simulink model "Vnernst"  (R2023a)
settings: Solver=VariableStepAuto  StartTime=0.0  StopTime=10.0  RelTol=1e-3
undefined symbols (not defined in the file): F, K, Kr, R, Uopt
settings Model: Creator=meghn  LastModifiedBy=meghn

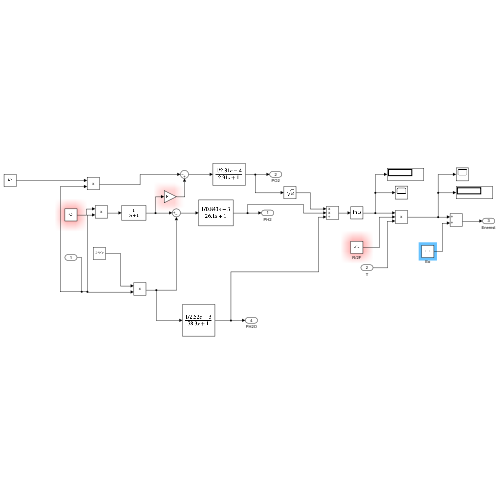
[thumbnail: Simulink's stored preview of the top-level diagram]
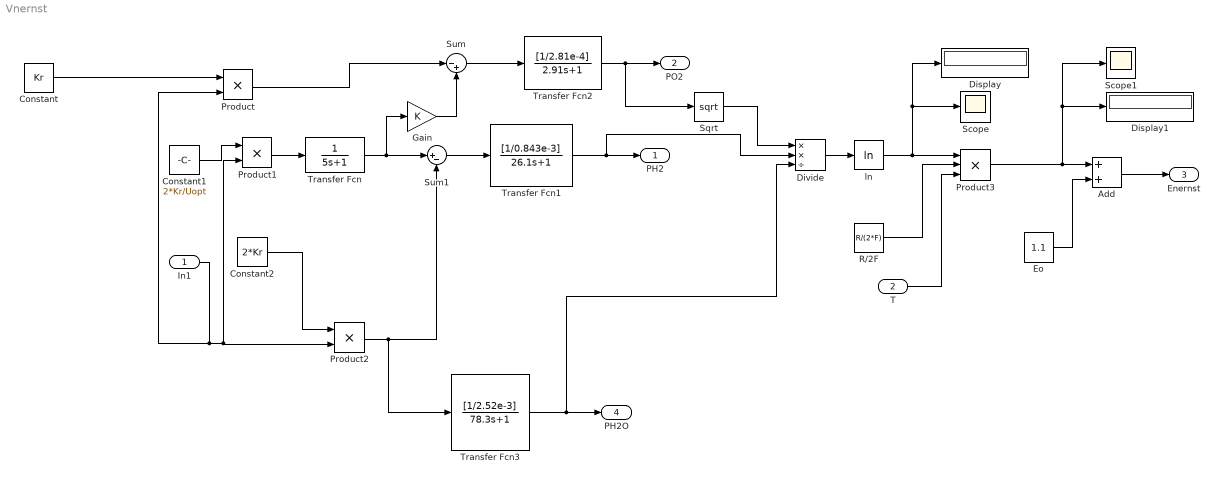
== system Vnernst ==
  In1 : Inport
  T : Inport  Port=2
  Add : Sum
  Constant : Constant  Value=Kr
  Constant1 : Constant  Value=2*Kr/Uopt
  Constant2 : Constant  Value=2*Kr
  Display : Display
  Display1 : Display
  Divide : Product  Inputs=**/
  Eo : Constant  Value=1.1
  Gain : Gain  Gain=K
  Product : Product
  Product1 : Product
  Product2 : Product
  Product3 : Product  Inputs=3
  R/2F : Constant  Value=R/(2*F)
  Scope : Scope
  Scope1 : Scope
  Sqrt : Sqrt
  Sum : Sum  Inputs=|-+
  Sum1 : Sum  Inputs=|+-
  Transfer Fcn : TransferFcn  Denominator=[5 1]
  Transfer Fcn1 : TransferFcn  Numerator=[1/0.843e-3]  Denominator=[26.1 1]
  Transfer Fcn2 : TransferFcn  Numerator=[1/2.81e-4]  Denominator=[2.91 1]
  Transfer Fcn3 : TransferFcn  Numerator=[1/2.52e-3]  Denominator=[78.3 1]
  ln : Math  Operator=log
  PH2 : Outport
  PO2 : Outport  Port=2
  Enernst : Outport  Port=3
  PH2O : Outport  Port=4
  wires:
  Constant/1 -> Product/1
  Constant1/1 -> Product1/1
  In1/1 -> Product1/2, Product2/2, Product/2
  Constant2/1 -> Product2/1
  Product1/1 -> Transfer Fcn/1
  Transfer Fcn/1 -> Gain/1, Sum1/1
  Product/1 -> Sum/1
  Gain/1 -> Sum/2
  Product2/1 -> Transfer Fcn3/1, Sum1/2
  Transfer Fcn3/1 -> Divide/3, PH2O/1
  Sum1/1 -> Transfer Fcn1/1
  Transfer Fcn1/1 -> Divide/2, PH2/1
  Sum/1 -> Transfer Fcn2/1
  Transfer Fcn2/1 -> Sqrt/1, PO2/1
  Sqrt/1 -> Divide/1
  Divide/1 -> ln/1
  ln/1 -> Product3/1, Scope/1, Display/1
  R/2F/1 -> Product3/2
  T/1 -> Product3/3
  Product3/1 -> Add/1, Scope1/1, Display1/1
  Eo/1 -> Add/2
  Add/1 -> Enernst/1
